simulink model "PMSM_PLLgaijin"  (R2018b)
settings: Solver=ode23  StartTime=0.0  StopTime=5  FixedStep=Ts  RelTol=1e-6  EnableMultiTasking=on
InitFcn:
  | Ts = 10e-6;
  | 
  | R = 0.958;
  | Ld = 12e-3;
  | Lq = 12e-3;
  | Pn = 4;
  | flux = 0.1827;
  | 
  | 
  | %Rs=140;Ld=.4;Lq=.4;Psai_r=.24;Pole=4;TL=.1;J=1e-3*2;B=.005;
  | %Udmax=150;Udc=500;ismax=2;
  | BASE_VOLTAGE=311/sqrt(3); %base peak phase votlage,Vdc/sqrt(3)
  | BASE_CURRENT=20; %base peak phase current
  | BASE_TORQUE=1;
  | BASE_FREQ=360; %240;     %Base electrical frequency (Hz)
  | BASE_FLUX=BASE_VOLTAGE/(2*pi*BASE_FREQ);   %Base flux linkage (volt.sec/rad)
  | 
  | Rs=0.958;Ld=12e-3;Lq=12e-3;Psai_r=0.1827;
  | Pole=4;TL=2;J=3.11e-4;B=0.001*10e-3;
  | 
  | Ts=1e-4;
  | Ts_pll=1e-3;
  | t_pll_on=3;
  | 
  | 
  | Target_fe = 300/BASE_FREQ;
  | 
  | %PLL
  | 
  | Ls=(Ld+Lq)/2
  | BW_PLL= 2*pi*20;
  | kesi_PLL= 1.7; %1.7;
  | Kp_PLL = 200;%2*kesi_PLL*BW_PLL;
  | Ki_PLL = 60;%BW_PLL*BW_PLL;
  | 
  | 
  | 
  | %current loop
  | BASE_Z=BASE_VOLTAGE/BASE_CURRENT;
  | Ld_pu=2*pi*Ld*BASE_FREQ/BASE_Z;
  | Lq_pu=2*pi*Lq*BASE_FREQ/BASE_Z;
  | Rs_pu=Rs/BASE_Z;
  | Psai_r_pu=Psai_r/BASE_FLUX
undefined symbols (not defined in the file): DiscIntNeverNeededParam
libraries: powerlib x4, powerlib_extras x2, simulink x1
settings Model: Creator=SUN  LastModifiedBy=liangjin
settings SolverCC: ZeroCrossControl=DisableAll  AlgebraicLoopSolver=LineSearch
settings DataIOCC: LimitDataPoints=on  SaveFormat=Array
settings OptimizationCC: ExpressionDepthLimit=2147483647  InitFltsAndDblsToZero=on  LifeSpan=inf
settings DebuggingCC: UnderspecifiedInitializationDetection=Classic  MergeDetectMultiDrivingBlocksExec=none  SolverPrmCheckMsg=warning  FcnCallInpInsideContextMsg=warning  StateNameClashWarn=warning  SFUnexpectedBacktrackingDiag=warning  SFNoUnconditionalDefaultTransitionDiag=warning  SFExecutionAtInitializationDiag=none
settings HardwareCC: ProdBitPerPointer=32  ProdBitPerSizeT=32  ProdBitPerPtrDiffT=32  ProdLargestAtomicFloat=None  ProdIntDivRoundTo=Undefined  ProdEndianess=Unspecified  ProdWordSize=32  ProdHWDeviceType=32-bit Generic
settings ModelReferenceCC: PropagateSignalLabelsOutOfModel=off
settings SFSimCC: SimUseLocalCustomCode=off
settings RTWCC: RTWUseLocalCustomCode=off
settings CodeAppCC: StateflowObjectComments=on
settings GRTTargetCC: TargetLangStandard=C89/C90 (ANSI)  GeneratePreprocessorConditionals=Disable all  CombineOutputUpdateFcns=off  GRTInterface=on
settings ConfigComp: CovMetricSettings=dw  CovHtmlReporting=on  CovSaveCumulativeToWorkspaceVar=on  CovSaveSingleToWorkspaceVar=on  CovExternalEMLEnable=off  CovSFcnEnable=off
settings SimscapeCC: SimscapeNormalizeSystem=off

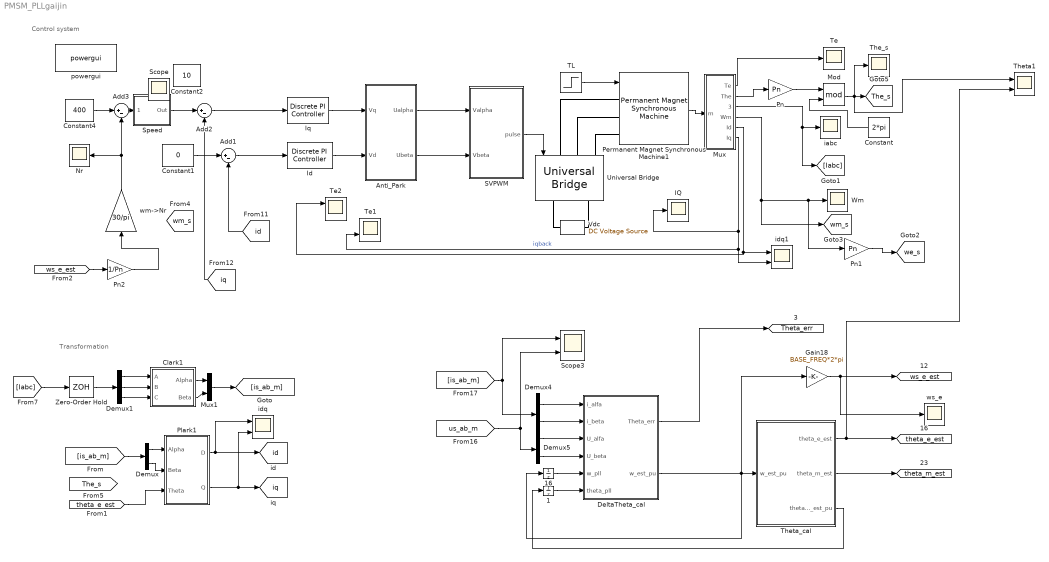
== system PMSM_PLLgaijin ==
  note: Control system
  note: Transformation
  " 1" : UnitDelay  SampleTime=Ts
  " 16" : UnitDelay  SampleTime=Ts
  " DeltaTheta_cal" : Subsystem
  Add1 : Sum  Inputs=|+-
  Add2 : Sum  Inputs=|+-
  Add3 : Sum  Inputs=|+-
  Anti_Park : Subsystem
  Clark1 : Subsystem
  Constant : Constant  Value=2*pi
  Constant1 : Constant  Value=0
  Constant2 : Constant  Value=10
  Constant4 : Constant  Value=400
  Demux : Demux  Outputs=2
  Demux1 : Demux  Outputs=3
  Demux4 : Demux  Outputs=2
  Demux5 : Demux  Outputs=2
  Gain18 : Gain  Gain=BASE_FREQ*2*pi
  IQ : Scope
  Id : powerlib_extras/Discrete  Control Blocks/Discrete PI Controller  Kp=Ld*0.11  Ki=R*0.125  Par_Limits=[311*0.9*sqrt(1/3) -311*0.9*sqrt(1/3)]  Init=0  Ts=Ts
  Iq : powerlib_extras/Discrete  Control Blocks/Discrete PI Controller  Kp=Lq*0.11  Ki=R*0.125  Par_Limits=[311*0.9*sqrt(1/3) -311*0.9*sqrt(1/3)]  Init=0  Ts=Ts
  Mod : Math  Operator=mod  SaturateOnIntegerOverflow=on
  Mux : Subsystem
  Mux1 : Mux  Inputs=2
  Nr : Scope
  Permanent Magnet Synchronous Machine1 : powerlib/Machines/Permanent Magnet Synchronous Machine  NbPhases=3  FluxDistribution=Sinusoidal  RotorType=Salient-pole  MechanicalLoad=Torque Tm  PresetModel=No  ShowDetailedParameters=on  MeasurementBus=off  Resistance=0.958  Inductance=8.5e-3  dqInductances=[12e-3,12e-3]  La=0.000835  MachineConstant=Flux linkage established by magnets (V.s)  Flux=0.1827  VoltageCst=132.5525  TorqueCst=1.0962  Flat=120  Mechanical=[0.001 0.01 4 0]  PolePairs=3  InitialConditions=[10,0, 0,0]  InitialConditions5ph=[0 0 0 0 0 0]  TsPowergui=0  TsBlock=-1  RefAngle=Aligned with phase A axis (original Park)
      settings: SourceProductName=Simscape Power Systems
  Plark1 : Subsystem
  Pn : Gain  Gain=Pn
  Pn1 : Gain  Gain=Pn
  Pn2 : Gain  Gain=1/Pn
  SVPWM : Subsystem
  Scope3 : Scope  NumInputPorts=2
  Speed : Subsystem  AncestorBlock=|  DialogController=POWERSYS.PowerSysDialog  mask(Discrete PI Controller){Kpw=0.045612, Kiw=0.045612*50, Ba=0, Par_Limits=[30 -30], Init=0, Ts=Ts}
      | powerlib_extras/Discrete 
      | Control Blocks/Discrete
      | PI Controller
      mask prompts: Kpw "Proportional gain (Kp):"; Kiw "Integral gain (Ki):"; Ba "feedback gain (Ba)"; Par_Limits "Output limits: [ Upper   Lower ]"; Init "Output initial value:"; Ts "Sample time:"
      mask help: This block implements a discrete PI controller.
      mask init:
      | UpperLimit=Par_Limits(1);
      | LowerLimit=Par_Limits(2);
      | power_initmask();
      mask Help: This block is part of a subset of blocks in the Extras library that does not have documentation associated with it, other than the block mask description.
      mask Display: disp('PI');
  TL : Step  Time=0  After=10  SampleTime=0
  Te : Scope
  Te1 : Scope  NumInputPorts=2
  Te2 : Scope  NumInputPorts=2
  The_s : Scope
  Theta1 : Scope  NumInputPorts=2
  Theta_cal : Subsystem
  Universal Bridge : powerlib/Power Electronics/Universal Bridge  Arms=3  SnubberResistance=1e5  SnubberCapacitance=inf  Device=IGBT / Diodes  Ron=1e-3  Lon=0  ForwardVoltages="[  0  0  ]"  ForwardVoltage=0  GTOparameters=[ 10e-6 , 20e-6 ]  IGBTparameters=[ 1e-6 , 2e-6 ]  Measurements=Device voltages  Measurements_2=None  converterType=Rectifier
  Vdc : powerlib/Electrical Sources/DC Voltage Source  Amplitude=311  Measurements=None
  Wm : Scope
  Zero-Order Hold : ZeroOrderHold  SampleTime=0.0001
  iabc : Scope
  idq : Scope  NumInputPorts=2
  idq1 : Scope  NumInputPorts=2
  powergui : powerlib/powergui  SimulationMode=Discrete  SampleTime=1e-05  frequency=60  Iterations=50  frequencyindice=0  Pbase=100e6  ErrMax=1e-4  UnitsV=kV  UnitsW=MW  buscounter=0  FunctionMessages=off  echomessages=off  EnableUseOfTLC=off  CurrentSourceSwitches=on  DisableSnubberDevices=off  DisableRonSwitches=off  DisableVfSwitches=off  DisplayEquations=off  SolverType=Tustin/Backward Euler (TBE)  Interpol=off  ExternalGateDelay=off  methode=off  Ts=0  x0status=blocks  SPID=off  SwTol=0  HookPort=off  RestoreLinks=warning  ResistiveCurrentMeasurement=off  Frange=[0:2:500]  Ylog=off  Xlog=on  ShowGrid=off  save=off  variable=ZData  structure=0  ZoomFFT=on  StartTime=0.0  cycles=1  DisplayStyle=1  fundamental=60  FreqAxis=off  MaxFrequency=1000  frequencyindicesteady=1  RmsSteady=1  display=off
  wm->Nr : Gain  Gain=30/pi
  ws_e : Scope
  Scope : Scope
  tag scope: The_s=global, Theta_err=global, id=global, iq=global, theta_e_est=global, theta_m_est=global, we_s=global, wm_s=global, ws_e_est=global
  wires:
  TL/1 -> Permanent Magnet Synchronous Machine1/1
  Permanent Magnet Synchronous Machine1/1 -> Mux/1(m)
  Constant1/1 -> Add1/1
  Add1/1 -> Id/1
  wm->Nr/1 -> Add3/2, Nr/1
  Iq/1 -> Anti_Park/1(Vq)
  Id/1 -> Anti_Park/2(Vd)
  Mux/1(Te) -> Te/1
  Mux/2(The) -> Pn/1
  SVPWM/1(pulse) -> Universal Bridge/1
  Demux1/1 -> Clark1/1(A)
  Demux1/2 -> Clark1/2(B)
  Demux1/3 -> Clark1/3(C)
  Clark1/1(Alpha) -> Mux1/1
  Clark1/2(Beta) -> Mux1/2
  Demux/1 -> Plark1/1(Alpha)
  Demux/2 -> Plark1/2(Beta)
  Anti_Park/1(Ualpha) -> SVPWM/1(Valpha)
  Anti_Park/2(Ubeta) -> SVPWM/2(Vbeta)
  Mux/3(Iabc) -> iabc/1, [Iabc]
  Constant4/1 -> Add3/1
  Add3/1 -> Speed/1(Error)
  Mux/4(Wm) -> Pn1/1, Wm/1, [wm_s]
  Constant/1 -> Mod/2
  Pn/1 -> Mod/1
  Mod/1 -> Theta1/1, [The_s], The_s/1
  Mux/5(Id) -> Te2/1, idq1/1
  Mux/6(Iq) -> idq1/2, Te1/2, IQ/1  "iqback"
  Theta_cal/1(theta_e_est) -> Theta1/2, [theta_e_est]
  [us_ab_m] -> Demux5/1, Scope3/2
  Gain18/1 -> ws_e/1, [ws_e_est]
  Theta_cal/2(theta_m_est) -> [theta_m_est]
  Theta_cal/3(theta_e_est_pu) -> " 1"/1
  Demux5/1 -> " DeltaTheta_cal"/3(U_alfa)
  " DeltaTheta_cal"/2(w_est_pu) -> Theta_cal/1(w_est_pu), Gain18/1, " 16"/1
  " DeltaTheta_cal"/1(Theta_err) -> [Theta_err]
  [is_ab_m] -> Demux4/1, Scope3/1
  Demux4/1 -> " DeltaTheta_cal"/1(i_alfa)
  Demux4/2 -> " DeltaTheta_cal"/2(i_beta)
  Demux5/2 -> " DeltaTheta_cal"/4(U_beta)
  Mux1/1 -> [is_ab_m]
  [is_ab_m] -> Demux/1
  Plark1/1(D) -> idq/1, [id]
  Plark1/2(Q) -> idq/2, [iq]
  Pn1/1 -> [we_s]
  " 16"/1 -> " DeltaTheta_cal"/5(w_pll)
  " 1"/1 -> " DeltaTheta_cal"/6(theta_pll)
  [Iabc] -> Zero-Order Hold/1
  Zero-Order Hold/1 -> Demux1/1
  [ws_e_est] -> Pn2/1
  Pn2/1 -> wm->Nr/1
  Add2/1 -> Iq/1
  [id] -> Add1/2
  [iq] -> Add2/2
  [theta_e_est] -> Plark1/3(Theta)
  Speed/1(Out) -> Add2/1
  connections:
  Universal Bridge/RConn1 -- Vdc/RConn1
  Universal Bridge/RConn2 -- Vdc/LConn1
  Permanent Magnet Synchronous Machine1/LConn1 -- Universal Bridge/LConn1
  Permanent Magnet Synchronous Machine1/LConn2 -- Universal Bridge/LConn2
  Permanent Magnet Synchronous Machine1/LConn3 -- Universal Bridge/LConn3

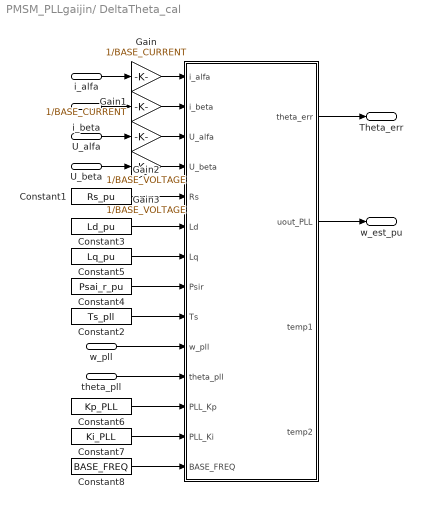
== system PMSM_PLLgaijin/ DeltaTheta_cal ==
  i_alfa : Inport
  i_beta : Inport  Port=2
  U_alfa : Inport  Port=3
  U_beta : Inport  Port=4
  w_pll : Inport  Port=5
  theta_pll : Inport  Port=6
  " " : MATLAB Function  TreatAsAtomicUnit=on
  Constant1 : Constant  Value=Rs_pu
  Constant2 : Constant  Value=Ts_pll
  Constant3 : Constant  Value=Ld_pu  VectorParams1D=off
  Constant4 : Constant  Value=Psai_r_pu  VectorParams1D=off
  Constant5 : Constant  Value=Lq_pu  VectorParams1D=off
  Constant6 : Constant  Value=Kp_PLL
  Constant7 : Constant  Value=Ki_PLL
  Constant8 : Constant  Value=BASE_FREQ
  Gain : Gain  Gain=1/BASE_CURRENT
  Gain1 : Gain  Gain=1/BASE_CURRENT
  Gain2 : Gain  Gain=1/BASE_VOLTAGE
  Gain3 : Gain  Gain=1/BASE_VOLTAGE
  Theta_err : Outport
  w_est_pu : Outport  Port=2
  wires:
  w_pll/1 -> " "/10(w_pll)
  U_beta/1 -> Gain3/1
  U_alfa/1 -> Gain2/1
  i_beta/1 -> Gain1/1
  i_alfa/1 -> Gain/1
  Constant1/1 -> " "/5(Rs)
  Constant3/1 -> " "/6(Ld)
  Constant2/1 -> " "/9(Ts)
  theta_pll/1 -> " "/11(theta_pll)
  Constant5/1 -> " "/7(Lq)
  " "/1(theta_err) -> Theta_err/1
  Constant4/1 -> " "/8(Psir)
  " "/2(uout_PLL) -> w_est_pu/1
  Constant6/1 -> " "/12(PLL_Kp)
  Constant7/1 -> " "/13(PLL_Ki)
  Constant8/1 -> " "/14(BASE_FREQ)
  Gain/1 -> " "/1(i_alfa)
  Gain1/1 -> " "/2(i_beta)
  Gain2/1 -> " "/3(U_alfa)
  Gain3/1 -> " "/4(U_beta)

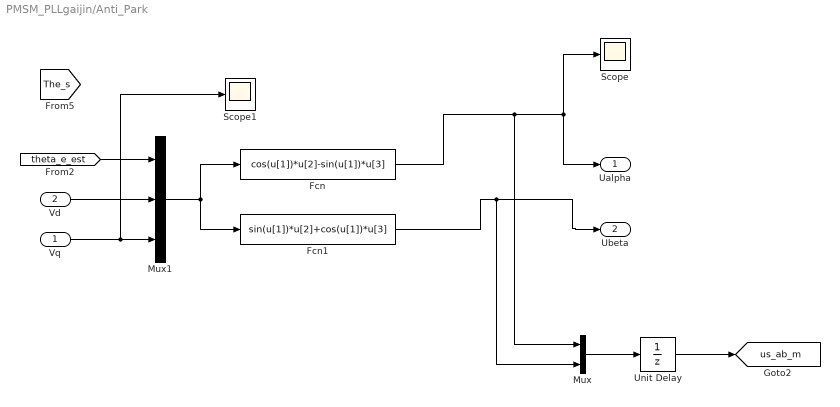
== system PMSM_PLLgaijin/Anti_Park ==
  Vq : Inport
  Vd : Inport  Port=2
  Fcn : Fcn  Expr=cos(u[1])*u[2]-sin(u[1])*u[3]
  Fcn1 : Fcn  Expr=sin(u[1])*u[2]+cos(u[1])*u[3]
  Mux : Mux  Inputs=2
  Mux1 : Mux  Inputs=3
  Scope : Scope
  Scope1 : Scope
  Unit Delay : UnitDelay  SampleTime=-1
  Ualpha : Outport
  Ubeta : Outport  Port=2
  tag scope: us_ab_m=global
  wires:
  Mux1/1 -> Fcn/1, Fcn1/1
  Vd/1 -> Mux1/2
  Vq/1 -> Scope1/1, Mux1/3
  Fcn/1 -> Mux/1, Scope/1, Ualpha/1
  Fcn1/1 -> Mux/2, Ubeta/1
  Mux/1 -> Unit Delay/1
  Unit Delay/1 -> [us_ab_m]
  [theta_e_est] -> Mux1/1

== system PMSM_PLLgaijin/Clark1 ==
  A : Inport
  B : Inport  Port=2
  C : Inport  Port=3
  Mux : Mux  Inputs=3
  alpha : Fcn  Expr=(u(1)-0.5*(u(2)+u(3)))*2/3
  beta : Fcn  Expr=sqrt(3)/2*(u(2)-u(3))*2/3
  Alpha : Outport
  Beta : Outport  Port=2
  wires:
  alpha/1 -> Alpha/1
  B/1 -> Mux/2
  C/1 -> Mux/3
  A/1 -> Mux/1
  Mux/1 -> beta/1, alpha/1
  beta/1 -> Beta/1

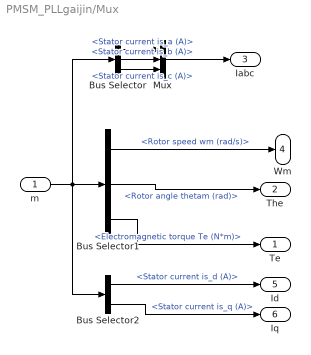
== system PMSM_PLLgaijin/Mux ==
  m : Inport
  Bus Selector : BusSelector  OutputSignals=Stator current is_a (A),Stator current is_b (A),Stator current is_c (A)
  Bus Selector1 : BusSelector  OutputSignals=Rotor speed wm (rad/s),Rotor angle thetam (rad),Electromagnetic torque Te (N*m)
  Bus Selector2 : BusSelector  OutputSignals=Stator current is_d (A),Stator current is_q (A)
  Mux : Mux  Inputs=3
  Te : Outport
  The : Outport  Port=2
  Iabc : Outport  Port=3
  Wm : Outport  Port=4
  Id : Outport  Port=5
  Iq : Outport  Port=6
  wires:
  Bus Selector1/1 -> Wm/1  "<Rotor speed wm (rad/s)>"
  Bus Selector1/2 -> The/1  "<Rotor angle thetam (rad)>"
  Bus Selector1/3 -> Te/1  "<Electromagnetic torque Te (N*m)>"
  m/1 -> Bus Selector2/1, Bus Selector/1, Bus Selector1/1
  Bus Selector/2 -> Mux/2  "<Stator current is_b (A)>"
  Bus Selector/3 -> Mux/3  "<Stator current is_c (A)>"
  Bus Selector/1 -> Mux/1  "<Stator current is_a (A)>"
  Mux/1 -> Iabc/1
  Bus Selector2/1 -> Id/1  "<Stator current is_d (A)>"
  Bus Selector2/2 -> Iq/1  "<Stator current is_q (A)>"

== system PMSM_PLLgaijin/Plark1 ==
  Alpha : Inport
  Beta : Inport  Port=2
  Theta : Inport  Port=3
  Mux : Mux  Inputs=3
  d : Fcn  Expr=u(1)*cos(u(3))+u(2)*sin(u(3))
  q : Fcn  Expr=-u(1)*sin(u(3))+u(2)*cos(u(3))
  D : Outport
  Q : Outport  Port=2
  wires:
  d/1 -> D/1
  Beta/1 -> Mux/2
  Alpha/1 -> Mux/1
  Mux/1 -> q/1, d/1
  q/1 -> Q/1
  Theta/1 -> Mux/3

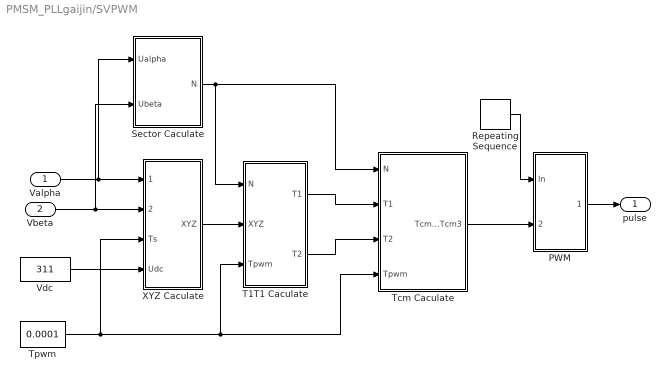
== system PMSM_PLLgaijin/SVPWM ==
  Valpha : Inport
  Vbeta : Inport  Port=2
  PWM : Subsystem
  Repeating Sequence : simulink/Sources/Repeating Sequence  rep_seq_t=[0 0.00005 0.0001]  rep_seq_y=[0 0.00005 0]
  Sector Caculate : Subsystem
  T1T1 Caculate : Subsystem
  Tcm Caculate : Subsystem
  Tpwm : Constant  Value=0.0001
  Vdc : Constant  Value=311
  XYZ Caculate : Subsystem
  pulse : Outport
  wires:
  PWM/1(PWM) -> pulse/1
  Repeating Sequence/1 -> PWM/1(In)
  T1T1 Caculate/1(T1) -> Tcm Caculate/2(T1)
  T1T1 Caculate/2(T2) -> Tcm Caculate/3(T2)
  Sector Caculate/1("N ") -> Tcm Caculate/1(N), T1T1 Caculate/1(N)
  XYZ Caculate/1(XYZ) -> T1T1 Caculate/2(XYZ)
  Tpwm/1 -> XYZ Caculate/3(Ts), Tcm Caculate/4(Tpwm), T1T1 Caculate/3(Tpwm)
  Vdc/1 -> XYZ Caculate/4(Udc)
  Tcm Caculate/1(Tcm1 Tcm2 Tcm3) -> PWM/2(Tcm123)
  Valpha/1 -> XYZ Caculate/1(Ualpha), Sector Caculate/1(Ualpha)
  Vbeta/1 -> XYZ Caculate/2(Ubeta), Sector Caculate/2(Ubeta)

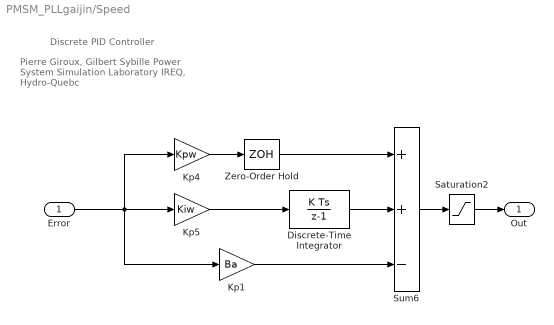
== system PMSM_PLLgaijin/Speed ==
  note: Discrete PID Controller
  note: Pierre Giroux, Gilbert Sybille
      | Power System Simulation Laboratory
      | IREQ, Hydro-Quebc
  Error : Inport  SampleTime=Ts
  Discrete-Time Integrator : DiscreteIntegrator  InitialCondition=Init  SampleTime=Ts  LimitOutput=on  UpperSaturationLimit=UpperLimit  LowerSaturationLimit=LowerLimit  ICPrevOutput=DiscIntNeverNeededParam  ICPrevScaledInput=DiscIntNeverNeededParam
  Kp1 : Gain  Gain=Ba  SampleTime=Ts  SaturateOnIntegerOverflow=on  OutDataTypeStr=Inherit: Same as input  ParamDataTypeStr=Inherit: Same as input
  Kp4 : Gain  Gain=Kpw  SampleTime=Ts  SaturateOnIntegerOverflow=on  OutDataTypeStr=Inherit: Same as input  ParamDataTypeStr=Inherit: Same as input
  Kp5 : Gain  Gain=Kiw  SampleTime=Ts  SaturateOnIntegerOverflow=on  OutDataTypeStr=Inherit: Same as input  ParamDataTypeStr=Inherit: Same as input
  Saturation2 : Saturate  UpperLimit=UpperLimit  LowerLimit=LowerLimit  SampleTime=Ts
  Sum6 : Sum  Inputs=++-  SampleTime=Ts  SaturateOnIntegerOverflow=on  InputSameDT=on  OutDataTypeStr=Inherit: Same as first input
  Zero-Order Hold : ZeroOrderHold  SampleTime=Ts
  Out : Outport  SampleTime=Ts  InitialOutput=0
  wires:
  Error/1 -> Kp1/1, Kp5/1, Kp4/1
  Zero-Order Hold/1 -> Sum6/1
  Saturation2/1 -> Out/1
  Discrete-Time Integrator/1 -> Sum6/2
  Kp4/1 -> Zero-Order Hold/1
  Kp5/1 -> Discrete-Time Integrator/1
  Sum6/1 -> Saturation2/1
  Kp1/1 -> Sum6/3

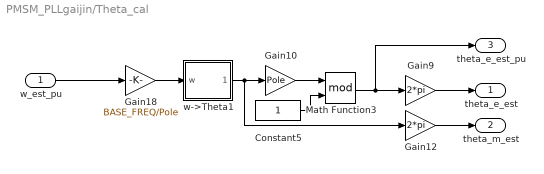
== system PMSM_PLLgaijin/Theta_cal ==
  w_est_pu : Inport
  Constant5 : Constant
  Gain10 : Gain  Gain=Pole
  Gain12 : Gain  Gain=2*pi
  Gain18 : Gain  Gain=BASE_FREQ/Pole
  Gain9 : Gain  Gain=2*pi
  Math Function3 : Math  Operator=mod  SaturateOnIntegerOverflow=on
  w->Theta1 : Subsystem
  theta_e_est : Outport
  theta_m_est : Outport  Port=2
  theta_e_est_pu : Outport  Port=3
  wires:
  Constant5/1 -> Math Function3/2
  Gain10/1 -> Math Function3/1
  Math Function3/1 -> theta_e_est_pu/1, Gain9/1
  Gain9/1 -> theta_e_est/1
  Gain12/1 -> theta_m_est/1
  Gain18/1 -> w->Theta1/1(w)
  w->Theta1/1(theta) -> Gain12/1, Gain10/1
  w_est_pu/1 -> Gain18/1

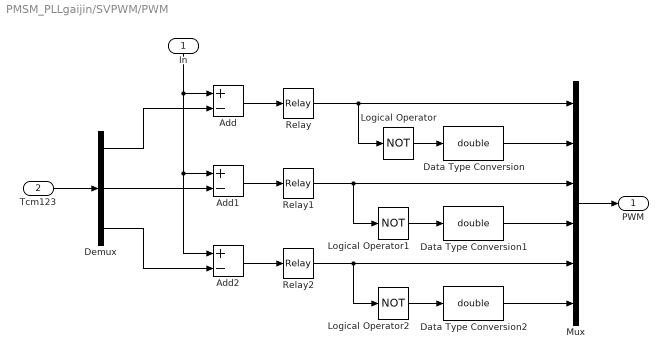
== system PMSM_PLLgaijin/SVPWM/PWM ==
  In : Inport
  Tcm123 : Inport  Port=2
  Add : Sum  Inputs=+-
  Add1 : Sum  Inputs=+-
  Add2 : Sum  Inputs=+-
  Data Type Conversion : DataTypeConversion  OutDataTypeStr=double
  Data Type Conversion1 : DataTypeConversion  OutDataTypeStr=double
  Data Type Conversion2 : DataTypeConversion  OutDataTypeStr=double
  Demux : Demux  Outputs=3
  Logical Operator : Logic  Operator=NOT  AllPortsSameDT=off  OutDataTypeStr=boolean
  Logical Operator1 : Logic  Operator=NOT  AllPortsSameDT=off  OutDataTypeStr=boolean
  Logical Operator2 : Logic  Operator=NOT  AllPortsSameDT=off  OutDataTypeStr=boolean
  Mux : Mux  Inputs=6
  Relay : Relay  OffSwitchValue=-eps
  Relay1 : Relay  OffSwitchValue=-eps
  Relay2 : Relay  OffSwitchValue=-eps
  PWM : Outport
  wires:
  Demux/3 -> Add2/2
  Demux/2 -> Add1/2
  Demux/1 -> Add/2
  Relay2/1 -> Mux/5, Logical Operator2/1
  Relay1/1 -> Mux/3, Logical Operator1/1
  Relay/1 -> Logical Operator/1, Mux/1
  Mux/1 -> PWM/1
  Data Type Conversion/1 -> Mux/2
  Data Type Conversion1/1 -> Mux/4
  Data Type Conversion2/1 -> Mux/6
  Logical Operator2/1 -> Data Type Conversion2/1
  Logical Operator1/1 -> Data Type Conversion1/1
  Logical Operator/1 -> Data Type Conversion/1
  Add1/1 -> Relay1/1
  Add2/1 -> Relay2/1
  Add/1 -> Relay/1
  In/1 -> Add/1, Add2/1, Add1/1
  Tcm123/1 -> Demux/1

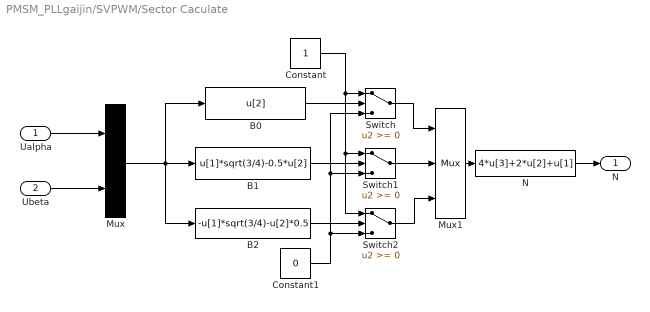
== system PMSM_PLLgaijin/SVPWM/Sector Caculate ==
  Ualpha : Inport
  Ubeta : Inport  Port=2
  B0 : Fcn  Expr=u[2]
  B1 : Fcn  Expr=u[1]*sqrt(3/4)-0.5*u[2]
  B2 : Fcn  Expr=-u[1]*sqrt(3/4)-u[2]*0.5
  Constant : Constant
  Constant1 : Constant  Value=0
  Mux : Mux  Inputs=2
  Mux1 : Mux  Inputs=3
  N : Fcn  Expr=4*u[3]+2*u[2]+u[1]
  Switch : Switch
  Switch1 : Switch
  Switch2 : Switch
  "N " : Outport
  wires:
  Switch2/1 -> Mux1/3
  Switch/1 -> Mux1/1
  Ualpha/1 -> Mux/1
  Ubeta/1 -> Mux/2
  Mux/1 -> B2/1, B1/1, B0/1
  B0/1 -> Switch/2
  B1/1 -> Switch1/2
  B2/1 -> Switch2/2
  Constant/1 -> Switch/1, Switch2/1, Switch1/1
  Constant1/1 -> Switch/3, Switch1/3, Switch2/3
  Switch1/1 -> Mux1/2
  Mux1/1 -> N/1
  N/1 -> "N "/1

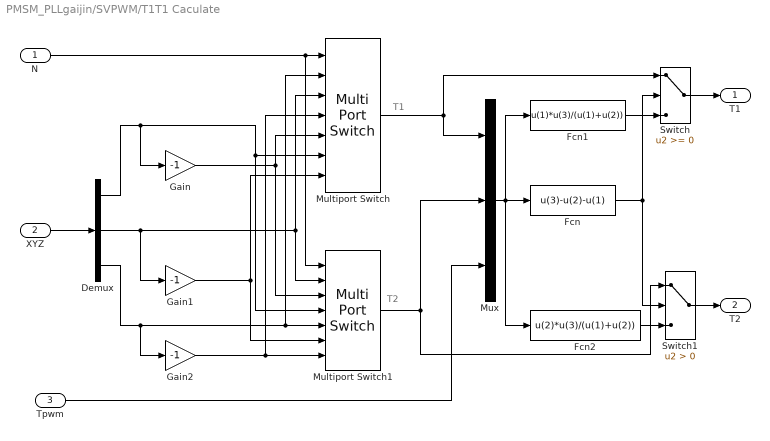
== system PMSM_PLLgaijin/SVPWM/T1T1 Caculate ==
  note: T1
  note: T2
  N : Inport
  XYZ : Inport  Port=2
  Tpwm : Inport  Port=3
  Demux : Demux  Outputs=3
  Fcn : Fcn  Expr=u(3)-u(2)-u(1)
  Fcn1 : Fcn  Expr=u(1)*u(3)/(u(1)+u(2))
  Fcn2 : Fcn  Expr=u(2)*u(3)/(u(1)+u(2))
  Gain : Gain  Gain=-1
  Gain1 : Gain  Gain=-1
  Gain2 : Gain  Gain=-1
  Multiport Switch : MultiPortSwitch  Inputs=6  DiagnosticForDefault=None
  Multiport Switch1 : MultiPortSwitch  Inputs=6  DiagnosticForDefault=None
  Mux : Mux  Inputs=3
  Switch : Switch
  Switch1 : Switch  Criteria=u2 > Threshold
  T1 : Outport
  T2 : Outport  Port=2
  wires:
  Tpwm/1 -> Mux/3
  XYZ/1 -> Demux/1
  Switch1/1 -> T2/1
  Switch/1 -> T1/1
  Fcn2/1 -> Switch1/3
  Fcn1/1 -> Switch/3
  Fcn/1 -> Switch/2, Switch1/2
  Mux/1 -> Fcn1/1, Fcn/1, Fcn2/1
  Multiport Switch/1 -> Switch/1, Mux/1
  Multiport Switch1/1 -> Switch1/1, Mux/2
  N/1 -> Multiport Switch/1, Multiport Switch1/1
  Demux/2 -> Multiport Switch/3, Multiport Switch1/2, Gain1/1
  Demux/3 -> Multiport Switch1/5, Multiport Switch/2, Gain2/1
  Demux/1 -> Multiport Switch/6, Multiport Switch1/4, Gain/1
  Gain/1 -> Multiport Switch1/3, Multiport Switch/5
  Gain2/1 -> Multiport Switch/4, Multiport Switch1/7
  Gain1/1 -> Multiport Switch1/6, Multiport Switch/7

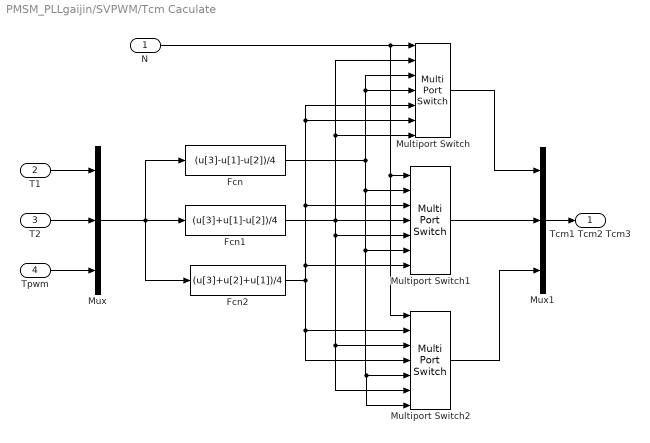
== system PMSM_PLLgaijin/SVPWM/Tcm Caculate ==
  N : Inport
  T1 : Inport  Port=2
  T2 : Inport  Port=3
  Tpwm : Inport  Port=4
  Fcn : Fcn  Expr=(u[3]-u[1]-u[2])/4
  Fcn1 : Fcn  Expr=(u[3]+u[1]-u[2])/4
  Fcn2 : Fcn  Expr=(u[3]+u[2]+u[1])/4
  Multiport Switch : MultiPortSwitch  Inputs=6  DiagnosticForDefault=None
  Multiport Switch1 : MultiPortSwitch  Inputs=6  DiagnosticForDefault=None
  Multiport Switch2 : MultiPortSwitch  Inputs=6  DiagnosticForDefault=None
  Mux : Mux  Inputs=3
  Mux1 : Mux  Inputs=3
  Tcm1 Tcm2 Tcm3 : Outport
  wires:
  Mux/1 -> Fcn2/1, Fcn/1, Fcn1/1
  Tpwm/1 -> Mux/3
  T2/1 -> Mux/2
  T1/1 -> Mux/1
  Multiport Switch2/1 -> Mux1/3
  Multiport Switch1/1 -> Mux1/2
  Multiport Switch/1 -> Mux1/1
  Mux1/1 -> Tcm1 Tcm2 Tcm3/1
  Fcn/1 -> Multiport Switch/3, Multiport Switch/4, Multiport Switch1/6, Multiport Switch2/5, Multiport Switch2/7, Multiport Switch1/2
  Fcn1/1 -> Multiport Switch1/5, Multiport Switch2/3, Multiport Switch2/6, Multiport Switch1/4, Multiport Switch/7, Multiport Switch/2
  Fcn2/1 -> Multiport Switch/5, Multiport Switch/6, Multiport Switch1/3, Multiport Switch1/7, Multiport Switch2/2, Multiport Switch2/4
  N/1 -> Multiport Switch2/1, Multiport Switch1/1, Multiport Switch/1

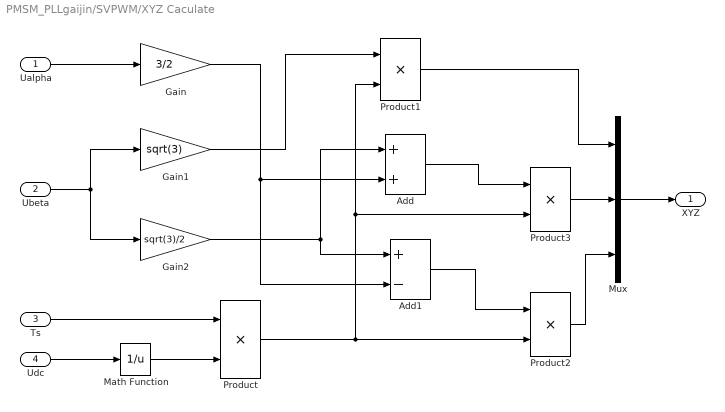
== system PMSM_PLLgaijin/SVPWM/XYZ Caculate ==
  Ualpha : Inport
  Ubeta : Inport  Port=2
  Ts : Inport  Port=3
  Udc : Inport  Port=4
  Add : Sum
  Add1 : Sum  Inputs=+-
  Gain : Gain  Gain=3/2
  Gain1 : Gain  Gain=sqrt(3)
  Gain2 : Gain  Gain=sqrt(3)/2
  Math Function : Math  Operator=reciprocal  SaturateOnIntegerOverflow=on
  Mux : Mux  Inputs=3
  Product{,1..3} (4 alike) : Product  RndMeth=Zero
  XYZ : Outport
  wires:
  Mux/1 -> XYZ/1
  Product1/1 -> Mux/1
  Product3/1 -> Mux/2
  Product2/1 -> Mux/3
  Ualpha/1 -> Gain/1
  Ubeta/1 -> Gain2/1, Gain1/1
  Udc/1 -> Math Function/1
  Math Function/1 -> Product/2
  Ts/1 -> Product/1
  Gain1/1 -> Product1/1
  Product/1 -> Product2/2, Product1/2, Product3/2
  Gain/1 -> Add1/2, Add/2
  Gain2/1 -> Add/1, Add1/1
  Add1/1 -> Product2/1
  Add/1 -> Product3/1

== system PMSM_PLLgaijin/Theta_cal/w->Theta1 ==
  w : Inport
  Constant2 : Constant
  Integrator1 : Integrator  ZeroCross=off
  Math Function3 : Math  Operator=mod  SaturateOnIntegerOverflow=on
  theta : Outport
  wires:
  Math Function3/1 -> theta/1
  w/1 -> Integrator1/1
  Constant2/1 -> Math Function3/2
  Integrator1/1 -> Math Function3/1

== matlab function PMSM_PLLgaijin/ DeltaTheta_cal/  ==
  settings: updateMethod=DISCRETE
  data: i_alfa input; i_beta input; U_alfa input; U_beta input; Rs input; Ld input; Lq input; Psir input; Ts input; w_pll input; theta_pll input; theta_err output; uout_PLL output; temp1 output; temp2 output; PLL_Kp input; PLL_Ki input; BASE_FREQ input
function [theta_err, uout_PLL,temp1,temp2]      = PLL2(i_alfa,i_beta,U_alfa,U_beta,Rs,Ld,Lq,Psir,Ts,w_pll,theta_pll,PLL_Kp,PLL_Ki,BASE_FREQ)


% refer 'Rolando' "Edsigh and Evaluation of PLL"
persistent id1 iq1 e_d_2  out_d ui_PLL w_pll_f;
if isempty(id1)    
   id1=0;iq1=0;e_d_2=0;out_d=0; ui_PLL=0;w_pll_f=0;
end
% U_alfa/beta -> Ud/q ,i_alfa/beta -> id/q
x1=theta_pll*2*pi;
Ud= cos(x1)*U_alfa+sin(x1)*U_beta;
Uq=-sin(x1)*U_alfa+cos(x1)*U_beta;
id= cos(x1)*i_alfa+sin(x1)*i_beta;
iq=-sin(x1)*i_alfa+cos(x1)*i_beta;

% Ud/q->ed/q(error theta)
%e_d=-(Ud-Rs*id-Ld*(id-id1)/Ts+w_pll*Lq*iq);
%e_q=  Uq-Rs*iq-Lq*(iq-iq1)/Ts-w_pll*Ld*id;

if 1
    id2=id;
    iq2=iq;
    
     w_pll_f =w_pll_f + 0.715*(w_pll-w_pll_f);

    e_d=(Ud-Rs*id2+w_pll_f*Lq*iq2);
%    e_mod=(Psir+(Ld-Lq)*id2)*w_pll_f;
    e_mod=(Psir)*w_pll_f;

    
    if (e_mod>-0.1 && e_mod<0)
        e_mod =-0.1;
    elseif (e_mod>=0 && e_mod<0.1)
        e_mod=0.1;
    end


    sin_=e_d/e_mod;

    if sin_>1
        sin_=1;
    elseif sin_<-1
        sin_=-1;
    end

        
    theta_err = -sin_;

   
    out_d = -sin_;


end


%save for next
id1=id;
iq1=iq;



% PI  for PLL
err_pll= theta_err/(2*pi*BASE_FREQ);
ui_PLL = PLL_Ki *err_pll*Ts+ ui_PLL;
uout_PLL = PLL_Kp*err_pll + ui_PLL;
if uout_PLL>1.2      uout_PLL=1.2;
elseif uout_PLL<0  uout_PLL=0;
end
ui_PLL =uout_PLL - PLL_Kp*err_pll;
if uout_PLL == 0
    ui_PLL=0;
end
%ui_PLL = uout_PLL-PLL_Kp*err_pll;

    temp1=e_d;
    temp2=e_mod;
